simulink model "fig10_71"  (Simulink 7.9)
settings: Solver=ode45  SolverMode=SingleTasking  StartTime=0.0  StopTime=170.0  RelTol=1e-6  AbsTol=1e-10
values from neighbouring files (symbols this model uses):
  A = [0    1.0000         0         0 ... (first row only)    [fig10_03.m]    (also in fig10_04.m; fig10_12.m; fig10_13.m; fig10_14.m)
  B = [0 ... (first row only)    [fig10_03.m]    (also in fig10_04.m; fig10_12.m; fig10_13.m; fig10_14.m)
  C = [1     0     0     0]    [fig10_03.m]    (also in fig10_04.m; fig10_12.m; fig10_13.m; fig10_14.m)
  L = place(A',C',pe)'    [fig10_21.m]    (also in fig10_22.m; fig10_23.m; fig10_24.m; fig10_37.m = place(Apw',Cpw',pe)')
undefined symbols (not defined in the file or in its folder): Conduction, InputFlux, K1, Ko, M_inv, Radiation, ScaleTemp
libraries: simulink x1
CloseFcn:
  | ;slview('closediagram',bdroot);
settings Model: Creator=abbas  LastModifiedBy=abbas  ExtModeTrigMode=oneshot  ExtModeArmWhenConnect=off
settings DataIOCC: LimitDataPoints=off
settings OptimizationCC: BlockReduction=off  BooleanDataType=off  InlineInvariantSignals=on  InitFltsAndDblsToZero=on
settings DebuggingCC: SaveWithParameterizedLinksMsg=none  SignalResolutionControl=TryResolveAllWithWarning  SolverPrmCheckMsg=none  MultiTaskDSMMsg=warning  MultiTaskCondExecSysMsg=none  FcnCallInpInsideContextMsg=Use local settings  StrictBusMsg=None
settings HardwareCC: TargetUnknown=on
settings RTWCC: IncludeERTFirstTime=on
settings GRTTargetCC: TargetFcnLib=ansi_tfl_tmw.mat  ModelReferenceCompliant=off  CompOptLevelCompliant=off  CombineOutputUpdateFcns=off  MatFileLogging=off  GRTInterface=on

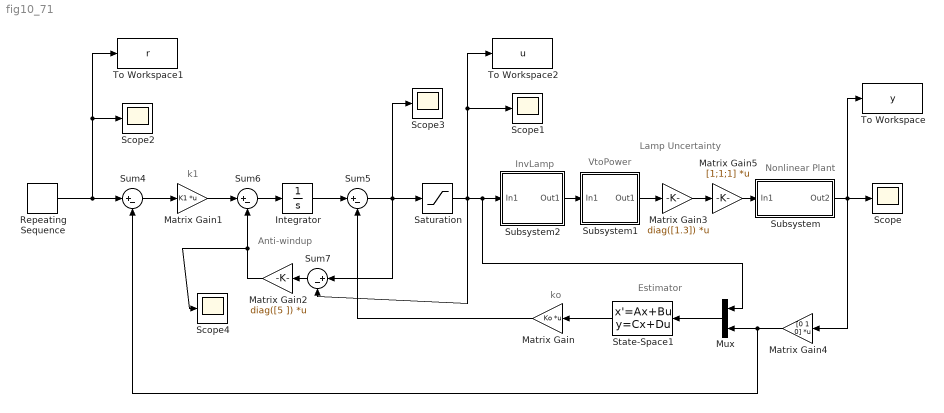
== system fig10_71 ==
  note: ko
  note: k1
  note: Nonlinear Plant
  note: InvLamp
  note: VtoPower
  note: Estimator
  note: Lamp
      | Uncertainty
  note: Anti-windup
  Integrator : Integrator
  Matrix Gain : Gain  Gain=Ko  Multiplication=Matrix(K*u)  SaturateOnIntegerOverflow=on  OutDataTypeStr=Inherit: Same as input  ParamDataTypeStr=Inherit: Same as input
  Matrix Gain1 : Gain  Gain=K1  Multiplication=Matrix(K*u)  SaturateOnIntegerOverflow=on  OutDataTypeStr=Inherit: Same as input  ParamDataTypeStr=Inherit: Same as input
  Matrix Gain2 : Gain  Gain=diag([5 ])  Multiplication=Matrix(K*u)  SaturateOnIntegerOverflow=on  OutDataTypeStr=Inherit: Same as input  ParamDataTypeStr=Inherit: Same as input
  Matrix Gain3 : Gain  Gain=diag([1.3])  Multiplication=Matrix(K*u)  SaturateOnIntegerOverflow=on  OutDataTypeStr=Inherit: Same as input  ParamDataTypeStr=Inherit: Same as input
  Matrix Gain4 : Gain  Gain=[0 1 0]  Multiplication=Matrix(K*u)  SaturateOnIntegerOverflow=on  OutDataTypeStr=Inherit: Same as input  ParamDataTypeStr=Inherit: Same as input
  Matrix Gain5 : Gain  Gain=[1;1;1]  Multiplication=Matrix(K*u)  SaturateOnIntegerOverflow=on  OutDataTypeStr=Inherit: Same as input  ParamDataTypeStr=Inherit: Same as input
  Mux : Mux  Inputs=2
  Repeating Sequence : simulink/Sources/Repeating Sequence  rep_seq_t=[0:0.1:170]  rep_seq_y="[313*ones(1,400) 313:.1:333 333*ones(1,400)  333:-.05:313 313*ones(1,299)]"
  Saturation : Saturate  UpperLimit=10  LowerLimit=0
  Scope{,1..4} (5 alike) : Scope
      settings: TickLabels=on
  State-Space1 : StateSpace  A=A-L*C  B=[B L]  C=eye(3)  D=0*ones(3,2)
  Subsystem : Subsystem
  Subsystem1 : Subsystem
  Subsystem2 : Subsystem
  Sum{4..7} (4 alike) : Sum  Inputs=|+-  SaturateOnIntegerOverflow=on  InputSameDT=on  OutDataTypeStr=Inherit: Same as first input
  To Workspace : ToWorkspace  VariableName=y  SampleTime=-1
  To Workspace1 : ToWorkspace  VariableName=r  SampleTime=-1
  To Workspace2 : ToWorkspace  VariableName=u  SampleTime=-1
  wires:
  Integrator/1 -> Sum5/1
  Saturation/1 -> Subsystem2/1(In1), Mux/1, Sum7/2, Scope1/1, To Workspace2/1
  Sum5/1 -> Saturation/1, Scope3/1, Sum7/1
  Subsystem2/1(Out1) -> Subsystem1/1(In1)
  Mux/1 -> State-Space1/1
  Subsystem/1(Out2) -> Scope/1, To Workspace/1, Matrix Gain4/1
  State-Space1/1 -> Matrix Gain/1
  Subsystem1/1(Out1) -> Matrix Gain3/1
  Sum4/1 -> Matrix Gain1/1
  Repeating Sequence/1 -> Sum4/1, Scope2/1, To Workspace1/1
  Matrix Gain/1 -> Sum5/2
  Sum6/1 -> Integrator/1
  Matrix Gain1/1 -> Sum6/1
  Sum7/1 -> Matrix Gain2/1
  Matrix Gain2/1 -> Sum6/2, Scope4/1
  Matrix Gain4/1 -> Mux/2, Sum4/2
  Matrix Gain3/1 -> Matrix Gain5/1
  Matrix Gain5/1 -> Subsystem/1(In1)

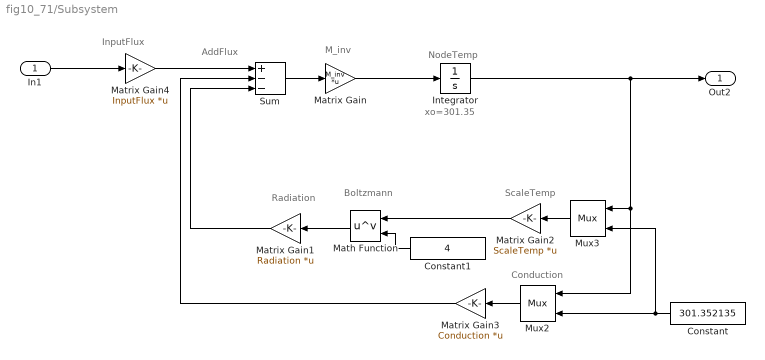
== system fig10_71/Subsystem ==
  note: InputFlux
  note: AddFlux
  note: M_inv
  note: NodeTemp
  note: xo=301.35
  note: Radiation
  note: ScaleTemp
  note: Conduction
  note: Boltzmann
  In1 : Inport
  Constant : Constant  Value=301.352135
  Constant1 : Constant  Value=4
  Integrator : Integrator  InitialCondition=301.3521350999999
  Math Function : Math  Operator=pow  SaturateOnIntegerOverflow=on
  Matrix Gain : Gain  Gain=M_inv  Multiplication=Matrix(K*u)  SaturateOnIntegerOverflow=on  OutDataTypeStr=Inherit: Same as input  ParamDataTypeStr=Inherit: Same as input
  Matrix Gain1 : Gain  Gain=Radiation  Multiplication=Matrix(K*u)  SaturateOnIntegerOverflow=on  OutDataTypeStr=Inherit: Same as input  ParamDataTypeStr=Inherit: Same as input
  Matrix Gain2 : Gain  Gain=ScaleTemp  Multiplication=Matrix(K*u)  SaturateOnIntegerOverflow=on  OutDataTypeStr=Inherit: Same as input  ParamDataTypeStr=Inherit: Same as input
  Matrix Gain3 : Gain  Gain=Conduction  Multiplication=Matrix(K*u)  SaturateOnIntegerOverflow=on  OutDataTypeStr=Inherit: Same as input  ParamDataTypeStr=Inherit: Same as input
  Matrix Gain4 : Gain  Gain=InputFlux  Multiplication=Matrix(K*u)  SaturateOnIntegerOverflow=on  OutDataTypeStr=Inherit: Same as input  ParamDataTypeStr=Inherit: Same as input
  Mux2 : Mux  Inputs=2
  Mux3 : Mux  Inputs=2
  Sum : Sum  Inputs=+--  SaturateOnIntegerOverflow=on  InputSameDT=on  OutDataTypeStr=Inherit: Same as first input
  Out2 : Outport
  wires:
  Matrix Gain4/1 -> Sum/1
  Sum/1 -> Matrix Gain/1
  Matrix Gain/1 -> Integrator/1
  Integrator/1 -> Mux2/1, Mux3/1, Out2/1
  Mux3/1 -> Matrix Gain2/1
  Mux2/1 -> Matrix Gain3/1
  Matrix Gain3/1 -> Sum/2
  Constant/1 -> Mux2/2, Mux3/2
  Matrix Gain1/1 -> Sum/3
  Math Function/1 -> Matrix Gain1/1
  Matrix Gain2/1 -> Math Function/1
  Constant1/1 -> Math Function/2
  In1/1 -> Matrix Gain4/1

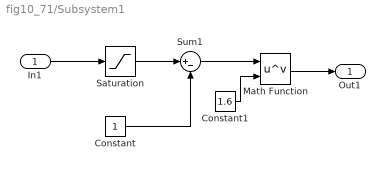
== system fig10_71/Subsystem1 ==
  In1 : Inport
  Constant : Constant
  Constant1 : Constant  Value=1.6
  Math Function : Math  Operator=pow  SaturateOnIntegerOverflow=on
  Saturation : Saturate  UpperLimit=4  LowerLimit=1
  Sum1 : Sum  Inputs=|+-  SaturateOnIntegerOverflow=on  InputSameDT=on  OutDataTypeStr=Inherit: Same as first input
  Out1 : Outport
  wires:
  In1/1 -> Saturation/1
  Saturation/1 -> Sum1/1
  Math Function/1 -> Out1/1
  Constant1/1 -> Math Function/2
  Sum1/1 -> Math Function/1
  Constant/1 -> Sum1/2

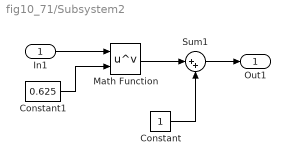
== system fig10_71/Subsystem2 ==
  In1 : Inport
  Constant : Constant
  Constant1 : Constant  Value=0.625
  Math Function : Math  Operator=pow  SaturateOnIntegerOverflow=on
  Sum1 : Sum  Inputs=|++  SaturateOnIntegerOverflow=on  InputSameDT=on  OutDataTypeStr=Inherit: Same as first input
  Out1 : Outport
  wires:
  In1/1 -> Math Function/1
  Math Function/1 -> Sum1/1
  Sum1/1 -> Out1/1
  Constant/1 -> Sum1/2
  Constant1/1 -> Math Function/2
